simulink model "SerialTest2018"  (R2018a)
settings: Solver=FixedStepAuto  StartTime=0.0  StopTime=inf  RelTol=1e-3  EnableMultiTasking=on
libraries: arduinolib x1, simulink x1
settings Model: ExtModeTrigDuration=2  Creator=Syed Imtiaz Ali Shah  LastModifiedBy=Syed Imtiaz Ali Shah
settings DataIOCC: ReturnWorkspaceOutputs=on
settings OptimizationCC: EnhancedBackFolding=on  PassReuseOutputArgsAs=Individual arguments  ZeroExternalMemoryAtStartup=off  ZeroInternalMemoryAtStartup=off  MaxStackSize=64  OptimizeBlockOrder=speed  DifferentSizesBufferReuse=on  OptimizationCustomize=off
settings DebuggingCC: ParameterTunabilityLossMsg=error  SFMachineParentedDataDiag=error
settings HardwareCC: ProdBitPerInt=16  ProdBitPerPointer=16  ProdBitPerSizeT=16  ProdBitPerPtrDiffT=16  ProdLargestAtomicFloat=None  ProdWordSize=8  ProdHWDeviceType=Atmel->AVR
settings SFSimCC: SimUseLocalCustomCode=on  MATLABDynamicMemAlloc=off
settings RTWCC: SystemTargetFile=ert.tlc  HardwareBoard=Arduino Mega 2560  TLCOptions=-aInlineSetEventsForThisBaseRateFcn=TLC_FALSE -aSuppressMultiTaskScheduler=TLC_FALSE -aRateBasedStepFcn=1  TemplateMakefile=ert_default_tmf  GenerateReport=on  RTWUseLocalCustomCode=on  Toolchain=Arduino AVR  BuildConfiguration=Faster Runs
settings CodeAppCC: ForceParamTrailComments=on  IgnoreCustomStorageClasses=off  OperatorAnnotations=on  SimulinkDataObjDesc=on  SFDataObjDesc=on  InsertBlockDesc=on
settings ERTTargetCC: SupportContinuousTime=on  SupportVariableSizeSignals=on  ExtModeTransport=3  ExtModeStaticAlloc=on  ExtModeStaticAllocSize=2048  ExtModeMexFile=ext_xcp  ExtModeIntrfLevel=Level2 - Open

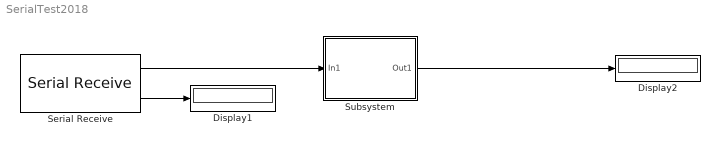
== system SerialTest2018 ==
  Display1 : Display
  Display2 : Display
  Serial Receive : arduinolib/Serial Receive  isARMArch=off  portNumber=1  DataType=uint8  Datalength=4  SampleTime=0.01  showOutStatus=on  blockPlatform=arduino
      settings: SourceProductBaseCode=ARDUINO
  Subsystem : Subsystem
      mask Display: image('C:\Users\Syed Imtiaz Ali Shah\Desktop\Capture.PNG'); % Use "Edit Image" on toolstrip to change.
  wires:
  Serial Receive/2 -> Display1/1
  Serial Receive/1 -> Subsystem/1(In1)
  Subsystem/1(Out1) -> Display2/1

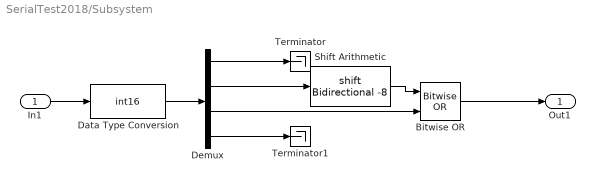
== system SerialTest2018/Subsystem ==
  In1 : Inport
  Bitwise OR : simulink/Logic and Bit Operations/Bitwise Operator  logicop=OR  UseBitMask=off  NumInputPorts=2  BitMask=bin2dec('11011001')  BitMaskRealWorld=Stored Integer
  Data Type Conversion : DataTypeConversion  OutDataTypeStr=int16
  Demux : Demux
  Shift Arithmetic : ArithShift  BitShiftNumber=-8
  Terminator : Terminator
  Terminator1 : Terminator
  Out1 : Outport
  wires:
  Shift Arithmetic/1 -> Bitwise OR/1
  Demux/1 -> Terminator/1
  Demux/3 -> Bitwise OR/2
  Demux/2 -> Shift Arithmetic/1
  Demux/4 -> Terminator1/1
  Bitwise OR/1 -> Out1/1
  Data Type Conversion/1 -> Demux/1
  In1/1 -> Data Type Conversion/1
